simulink model "jiang"  (R2016a)
settings: Solver=FixedStepAuto  StartTime=0.0  StopTime=1000  FixedStep=0.05  RelTol=1e-3
libraries: simulink x2
settings Model: Creator=Staciej  LastModifiedBy=Staciej

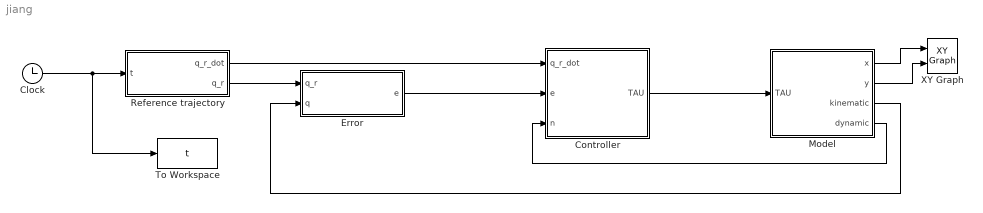
== system jiang ==
  Clock : Clock
  Controller : Subsystem
  Error : Subsystem
  Model : Subsystem
  Reference trajectory : Subsystem
  To Workspace : ToWorkspace  VariableName=t  SampleTime=-1
  XY Graph : simulink/Sinks/XY Graph  xmin=-100  xmax=1000  ymin=-200  ymax=200  st=-1
  wires:
  Clock/1 -> To Workspace/1, Reference trajectory/1(t)
  Controller/1(TAU) -> Model/1(TAU)
  Model/1(x) -> XY Graph/1
  Model/2(y) -> XY Graph/2
  Reference trajectory/2(q_r) -> Error/1(q_r)
  Error/1(e) -> Controller/2(e)
  Model/4(dynamic) -> Controller/3(n)
  Model/3(kinematic) -> Error/2(q)
  Reference trajectory/1(q_r_dot) -> Controller/1(q_r_dot)

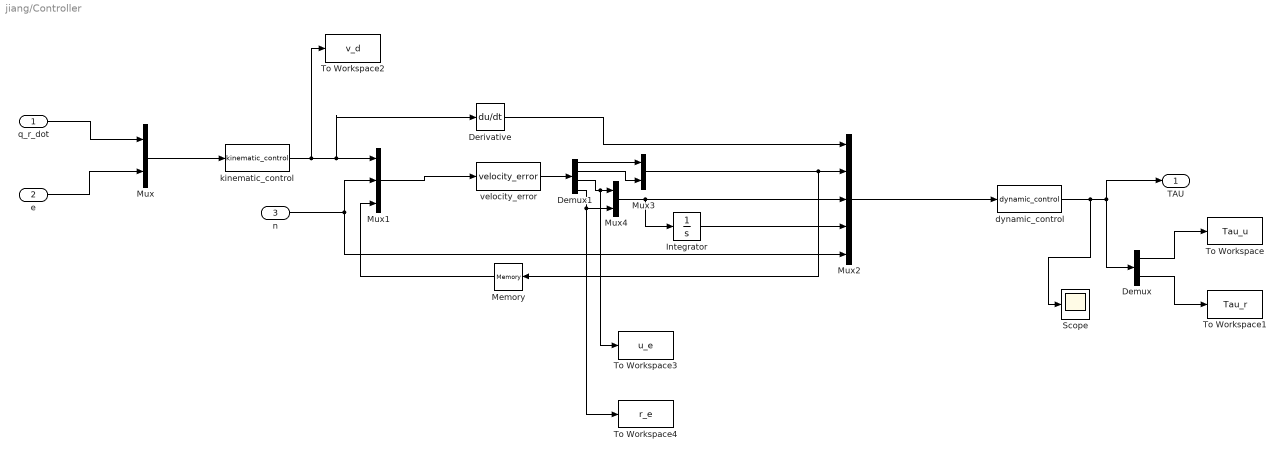
== system jiang/Controller ==
  q_r_dot : Inport
  e : Inport  Port=2
  n : Inport  Port=3
  Demux : Demux  Outputs=2
  Demux1 : Demux
  Derivative : Derivative
  Integrator : Integrator
  Memory : Memory  X0=[0;0]
  Mux : Mux  Inputs=2
  Mux1 : Mux  Inputs=3
  Mux2 : Mux  Inputs=5
  Mux3 : Mux  Inputs=2
  Mux4 : Mux  Inputs=2
  Scope : Scope
  To Workspace : ToWorkspace  VariableName=Tau_u  SampleTime=-1
  To Workspace1 : ToWorkspace  VariableName=Tau_r  SampleTime=-1
  To Workspace2 : ToWorkspace  VariableName=v_d  SampleTime=-1
  To Workspace3 : ToWorkspace  VariableName=u_e  SampleTime=-1
  To Workspace4 : ToWorkspace  VariableName=r_e  SampleTime=-1
  dynamic_control : MATLABFcn  MATLABFcn=dynamic_control  OutputDimensions=2
  kinematic_control : MATLABFcn  MATLABFcn=kinematic_control  OutputDimensions=2
  velocity_error : MATLABFcn  MATLABFcn=velocity_error  OutputDimensions=4
  TAU : Outport
  wires:
  dynamic_control/1 -> Scope/1, Demux/1, TAU/1
  Demux/1 -> To Workspace/1
  Demux/2 -> To Workspace1/1
  q_r_dot/1 -> Mux/1
  e/1 -> Mux/2
  Mux/1 -> kinematic_control/1
  kinematic_control/1 -> To Workspace2/1, Derivative/1, Mux1/1
  Mux1/1 -> velocity_error/1
  n/1 -> Mux1/2, Mux2/5
  velocity_error/1 -> Demux1/1
  Demux1/1 -> Mux3/1
  Demux1/2 -> Mux3/2
  Mux3/1 -> Memory/1, Mux2/2
  Demux1/3 -> To Workspace3/1, Mux4/1
  Demux1/4 -> To Workspace4/1, Mux4/2
  Mux4/1 -> Mux2/3, Integrator/1
  Integrator/1 -> Mux2/4
  Derivative/1 -> Mux2/1
  Mux2/1 -> dynamic_control/1
  Memory/1 -> Mux1/3

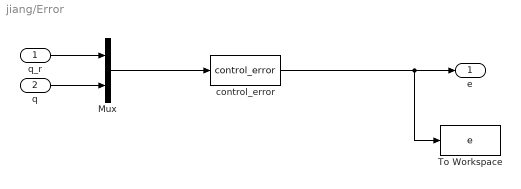
== system jiang/Error ==
  q_r : Inport
  q : Inport  Port=2
  Mux : Mux  Inputs=2
  To Workspace : ToWorkspace  VariableName=e  SampleTime=-1
  control_error : MATLABFcn  MATLABFcn=control_error  OutputDimensions=3
  e : Outport
  wires:
  q_r/1 -> Mux/1
  Mux/1 -> control_error/1
  q/1 -> Mux/2
  control_error/1 -> To Workspace/1, e/1

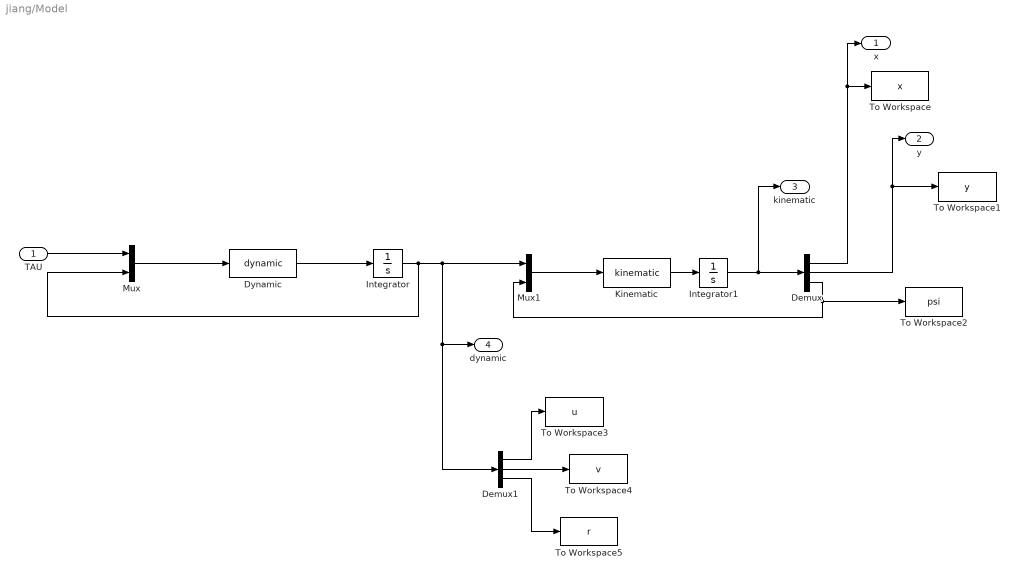
== system jiang/Model ==
  TAU : Inport
  Demux : Demux  Outputs=3
  Demux1 : Demux  Outputs=3
  Dynamic : MATLABFcn  MATLABFcn=dynamic  OutputDimensions=3
  Integrator : Integrator  InitialCondition=[0 0 0]
  Integrator1 : Integrator  InitialCondition=[5 10 0.5]
  Kinematic : MATLABFcn  MATLABFcn=kinematic  OutputDimensions=3
  Mux : Mux  Inputs=2
  Mux1 : Mux  Inputs=2
  To Workspace : ToWorkspace  VariableName=x  SampleTime=-1
  To Workspace1 : ToWorkspace  VariableName=y  SampleTime=-1
  To Workspace2 : ToWorkspace  VariableName=psi  SampleTime=-1
  To Workspace3 : ToWorkspace  VariableName=u  SampleTime=-1
  To Workspace4 : ToWorkspace  VariableName=v  SampleTime=-1
  To Workspace5 : ToWorkspace  VariableName=r  SampleTime=-1
  x : Outport
  y : Outport  Port=2
  kinematic : Outport  Port=3
  dynamic : Outport  Port=4
  wires:
  TAU/1 -> Mux/1
  Mux/1 -> Dynamic/1
  Dynamic/1 -> Integrator/1
  Integrator/1 -> Mux/2, Demux1/1, dynamic/1, Mux1/1
  Mux1/1 -> Kinematic/1
  Kinematic/1 -> Integrator1/1
  Demux/3 -> To Workspace2/1, Mux1/2
  Demux/1 -> x/1, To Workspace/1
  Demux/2 -> y/1, To Workspace1/1
  Integrator1/1 -> kinematic/1, Demux/1
  Demux1/1 -> To Workspace3/1
  Demux1/2 -> To Workspace4/1
  Demux1/3 -> To Workspace5/1

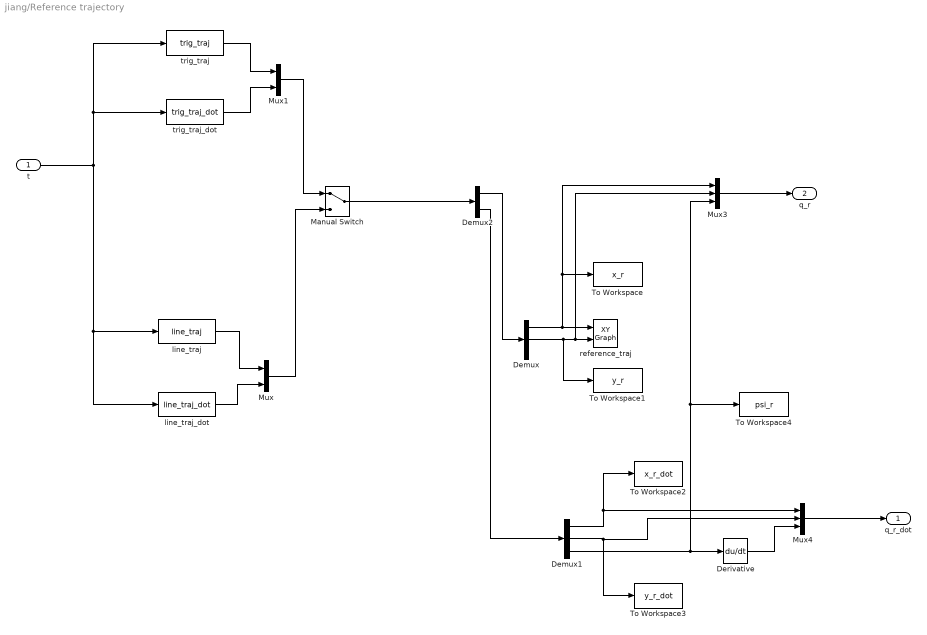
== system jiang/Reference trajectory ==
  t : Inport
  Demux : Demux  Outputs=3
  Demux1 : Demux  Outputs=3
  Demux2 : Demux  Outputs=2
  Derivative : Derivative
  Manual Switch : ManualSwitch
  Mux : Mux  Inputs=2
  Mux1 : Mux  Inputs=2
  Mux3 : Mux  Inputs=3
  Mux4 : Mux  Inputs=3
  To Workspace : ToWorkspace  VariableName=x_r  SampleTime=-1
  To Workspace1 : ToWorkspace  VariableName=y_r  SampleTime=-1
  To Workspace2 : ToWorkspace  VariableName=x_r_dot  SampleTime=-1
  To Workspace3 : ToWorkspace  VariableName=y_r_dot  SampleTime=-1
  To Workspace4 : ToWorkspace  VariableName=psi_r  SampleTime=-1
  line_traj : MATLABFcn  MATLABFcn=line_traj  OutputDimensions=3
  line_traj_dot : MATLABFcn  MATLABFcn=line_traj_dot  OutputDimensions=3
  reference_traj : simulink/Sinks/XY Graph  xmin=-100  xmax=1000  ymin=-200  ymax=200  st=-1
  trig_traj : MATLABFcn  MATLABFcn=trig_traj  OutputDimensions=3
  trig_traj_dot : MATLABFcn  MATLABFcn=trig_traj_dot  OutputDimensions=3
  q_r_dot : Outport
  q_r : Outport  Port=2
  wires:
  t/1 -> trig_traj_dot/1, trig_traj/1, line_traj/1, line_traj_dot/1
  Demux/1 -> Mux3/1, To Workspace/1, reference_traj/1
  Demux/2 -> To Workspace1/1, Mux3/2, reference_traj/2
  Demux1/1 -> Mux4/1, To Workspace2/1
  Demux1/2 -> Mux4/2, To Workspace3/1
  Demux2/2 -> Demux1/1
  line_traj_dot/1 -> Mux/2
  line_traj/1 -> Mux/1
  Mux/1 -> Manual Switch/2
  Demux2/1 -> Demux/1
  trig_traj_dot/1 -> Mux1/2
  trig_traj/1 -> Mux1/1
  Mux1/1 -> Manual Switch/1
  Manual Switch/1 -> Demux2/1
  Demux1/3 -> Derivative/1, To Workspace4/1, Mux3/3
  Derivative/1 -> Mux4/3
  Mux4/1 -> q_r_dot/1
  Mux3/1 -> q_r/1
